simulink model "task4"  (R2020a)
settings: Solver=VariableStepAuto  StartTime=0.0  StopTime=tf  RelTol=1e-3
values from neighbouring files (symbols this model uses):
  Kd = 50    [task4_script.m]
  Kp = 100    [task4_script.m]
libraries: roblocks x4
settings Model: Creator=root  LastModifiedBy=root

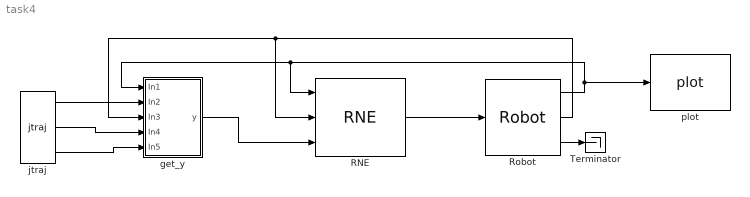
== system task4 ==
  RNE : roblocks/Arm/RNE  robot=p560Unc  grav=[0 0 9.81]
  Robot : roblocks/Arm/Robot  robot=p560  q0=[0 0 0 0 0 0]
  Terminator : Terminator
  get_y : Subsystem
  jtraj : roblocks/Toolbox/jtraj  q0=qz  qf=qr  tmax=5.0  ts=0.02
  plot : roblocks/Arm/plot  robot=p560  fps=5  holdplot=on
  wires:
  Robot/1 -> plot/1, get_y/1(In1), RNE/1
  jtraj/1 -> get_y/2(In2)
  Robot/2 -> get_y/3(In3), RNE/2
  jtraj/2 -> get_y/4(In4)
  jtraj/3 -> get_y/5(In5)
  get_y/1(y) -> RNE/3
  RNE/1 -> Robot/1
  Robot/3 -> Terminator/1

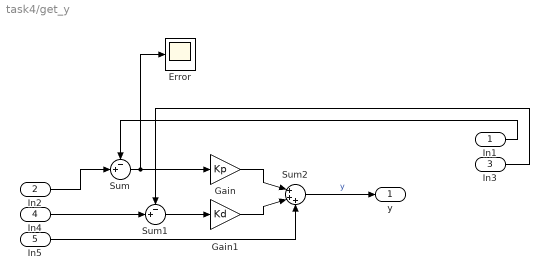
== system task4/get_y ==
  In1 : Inport
  In2 : Inport  Port=2
  In3 : Inport  Port=3
  In4 : Inport  Port=4
  In5 : Inport  Port=5
  Error : Scope
  Gain : Gain  Gain=Kp
  Gain1 : Gain  Gain=Kd
  Sum : Sum  Inputs=-+|
  Sum1 : Sum  Inputs=-+|
  Sum2 : Sum  Inputs=|+++
  y : Outport
  wires:
  Sum/1 -> Error/1, Gain/1
  In1/1 -> Sum/1
  Gain1/1 -> Sum2/2
  In5/1 -> Sum2/3
  Gain/1 -> Sum2/1
  In2/1 -> Sum/2
  Sum2/1 -> y/1  "y"
  Sum1/1 -> Gain1/1
  In4/1 -> Sum1/2
  In3/1 -> Sum1/1
